simulink model "mdl_4reac"  (R2020b)
settings: Solver=FixedStepAuto  StartTime=0.0  StopTime=stoptime  FixedStep=0.001  MaxStep=1  RelTol=1e-3  AbsTol=1e-6
undefined symbols (not defined in the file or in its folder): p, ref_select, strategy_select
(part 2 of 2)

== stateflow chart mdl_4reac/2 pumps interval strategy ==
  state counter_inflow [parallel]
    settings: executionOrder=1
    state init_counter
      entry: reac_ind_inflow = 1;
    state increase_counter
      entry: reac_ind_inflow = reac_ind_inflow+1;
    state cycle_over
    (default) -> counter_inflow.init_counter : % loop_counter
    (junction 211) -> counter_inflow.cycle_over [order 2]
    (junction 211) -> counter_inflow.increase_counter [order 1] : [reac_ind_inflow<p.num_reac]
    counter_inflow.increase_counter -> (junction 211) : after(p.interval/p.num_reac,sec)
    counter_inflow.init_counter -> counter_inflow.increase_counter : after(p.interval/p.num_reac,sec)
    counter_inflow.cycle_over -> counter_inflow.init_counter
  state counter_outflow [parallel]
    settings: executionOrder=4
    state init_counter
      entry: reac_ind_outflow = 1;
    state increase_counter
      entry: reac_ind_outflow = reac_ind_outflow+1;
    state cycle_over
    (default) -> counter_outflow.init_counter : % loop_counter
    (junction 274) -> counter_outflow.cycle_over [order 2]
    (junction 274) -> counter_outflow.increase_counter [order 1] : [reac_ind_outflow<p.num_reac]
    counter_outflow.increase_counter -> (junction 274) : after(p.interval/p.num_reac,sec)
    counter_outflow.init_counter -> counter_outflow.increase_counter : after(p.interval/p.num_reac,sec)
    counter_outflow.cycle_over -> counter_outflow.init_counter : next_cycle
  state procedures [parallel]
    settings: executionOrder=3
    state normal
    state sampling
      entry: sampling_req=true;
    (default) -> normal
    normal -> sampling : after(15, sec)
    sampling -> normal : sampling_done
  state feeding [parallel]
    settings: executionOrder=5
    state inflow
      state inflow_act
        entry: vol_pump_in=floor(des_vol(reac_ind_inflow)/...
        p.pump_res)*p.pump_res;
        act_pump_inflow(reac_ind_inflow)=p.max_pump_flow;
      state inflow_inact
        entry: act_pump_inflow=zeros(4,1);
      inflow_act -> inflow_inact [order 3] : [vol_pump_in<=0]
      inflow_act -> inflow_inact [order 1] : after(vol_pump_in/p.max_pump_flow,sec)
      inflow_inact -> inflow_act [order 1] : enter(counter_inflow.increase_counter)
      inflow_inact -> inflow_act [order 2] : enter(counter_inflow.init_counter)
      inflow_act -> inflow_inact [order 2] : after(p.interval/p.num_reac-1e-3,sec)
    (default) -> inflow_act
  state wasting_sampling [parallel]
    settings: executionOrder=2
    state outflow_waste
      state outflow_act
        entry:vol_pump_out = reactor_vol(reac_ind_outflow);
        %vol_pump_out=...
        %  floor(reactor_vol(reac_ind_outflow)/...
        %  p.pump_res)*p.pump_res;
        act_pump_outflow(reac_ind_outflow)=p.max_pump_flow;
      state outflow_inact
        entry: act_pump_outflow=zeros(4,1);
      wasting_sampling.outflow_waste.outflow_inact -> wasting_sampling.outflow_waste.outflow_act [order 1] : [enter(counter_outflow.cycle_over) && in(procedures.normal)]{send(next_cycle,counter_outflow)}
      wasting_sampling.outflow_waste.outflow_act -> wasting_sampling.outflow_waste.outflow_inact [order 1] : [vol_pump_out<=0]
      wasting_sampling.outflow_waste.outflow_act -> wasting_sampling.outflow_waste.outflow_inact [order 2] : after(vol_pump_out/p.max_pump_flow,sec)
      wasting_sampling.outflow_waste.outflow_inact -> wasting_sampling.outflow_waste.outflow_act [order 2] : enter(counter_outflow.increase_counter)
      wasting_sampling.outflow_waste.outflow_act -> wasting_sampling.outflow_waste.outflow_inact [order 3] : after(p.interval/p.num_reac-1e-3,sec)
    state cleaning_procedure
    state outflow_sampling
      state outflow_act
        entry: vol_pump_out=p.pump_res;
        act_pump_outflow(reac_ind_outflow)=...
        p.max_pump_flow;
      state outflow_inact
        entry: act_pump_outflow=zeros(4,1);
      wasting_sampling.outflow_sampling.outflow_act -> wasting_sampling.outflow_sampling.outflow_inact : after(vol_pump_out/p.max_pump_flow,sec)
      wasting_sampling.outflow_sampling.outflow_inact -> wasting_sampling.outflow_sampling.outflow_act [order 1] : enter(counter_outflow.increase_counter)
    (default) -> wasting_sampling.outflow_waste.outflow_act
    wasting_sampling.outflow_waste.outflow_inact -> cleaning_procedure [order 3] : [enter(counter_outflow.cycle_over) && in(procedures.sampling)]
    wasting_sampling.outflow_sampling.outflow_inact -> wasting_sampling.outflow_waste.outflow_act [order 2] : [enter(counter_outflow.cycle_over)]{send(sampling_done, procedures);send(next_cycle, counter_outflow)}
    cleaning_procedure -> (junction 263) : after(p.clean_time,sec)
    (junction 263) -> wasting_sampling.outflow_sampling.outflow_act : {send(next_cycle,counter_outflow)}
  data: act_pump_inflow output =[0;0;0;0]; reactor_vol input; des_vol input size=4; vol_pump_in local; act_pump_outflow output =[0;0;0;0]; vol_pump_out local; reac_ind_inflow local =1; sampling_req local; p parameter; reac_ind_outflow local =1
  events: sampling_done local FUNCTION_CALL_EVENT; next_cycle local FUNCTION_CALL_EVENT
